simulink model "ThdRwLtStCshnFldTrgtPosSelc"  (R2018b)
settings: Solver=FixedStepDiscrete  StartTime=0.0  StopTime=10.0  RelTol=1e-3
undefined symbols (not defined in the file or in its folder): KeSMSw6sAcsEntryThdRwLtStCshnFldUpwdDnwdPos_Val, KeSMSw6sAcsEntryThdRwLtStCshnFldUpwdDnwdPosMax_Val, KeSMSw6sAcsEntryThdRwLtStCshnFldUpwdDnwdPosMin_Val, KeSMSw6sLugThdRwLtStCshnFldUpwdDnwdPos_Val, KeSMSw6sLugThdRwLtStCshnFldUpwdDnwdPosMax_Val, KeSMSw6sLugThdRwLtStCshnFldUpwdDnwdPosMin_Val, KeSMSwAcsEntryThdRwLtStCshnFldUpwdDnwdPos_Val, KeSMSwAcsEntryThdRwLtStCshnFldUpwdDnwdPosMax_Val, KeSMSwAcsEntryThdRwLtStCshnFldUpwdDnwdPosMin_Val, KeSMSwAcsMd32ThdRwLtFldUpwdDnwdPos_Val, KeSMSwAcsMd32ThdRwLtFldUpwdDnwdPosMax_Val, KeSMSwAcsMd32ThdRwLtFldUpwdDnwdPosMin_Val, KeSMSwLugThdRwLtStCshnFldUpwdDnwdPos_Val, KeSMSwLugThdRwLtStCshnFldUpwdDnwdPosMax_Val, KeSMSwLugThdRwLtStCshnFldUpwdDnwdPosMin_Val
libraries: TrgtPosSelcLib x4
settings Model: ModifiedHistory=2024.6.25 V2.1.0 557模式流程V1.6  Creator=sn2xws  LastModifiedBy=sn2xws
settings DataIOCC: SaveFormat=StructureWithTime
settings OptimizationCC: DefaultParameterBehavior=Inlined  EnhancedBackFolding=on  PassReuseOutputArgsAs=Individual arguments  ZeroExternalMemoryAtStartup=off  ZeroInternalMemoryAtStartup=off  OptimizeBlockOrder=speed  DifferentSizesBufferReuse=on  OptimizationCustomize=off
settings DebuggingCC: ParameterTunabilityLossMsg=error
settings SFSimCC: MATLABDynamicMemAlloc=off
settings RTWCC: SystemTargetFile=autosar.tlc  GenCodeOnly=on  TemplateMakefile=ert_default_tmf  Description=AUTOSAR  GenerateReport=on  IncludeHyperlinkInReport=on  LaunchReport=on  GenerateTraceInfo=on  GenerateTraceReport=on  GenerateTraceReportSl=on  GenerateTraceReportSf=on  GenerateTraceReportEml=on
settings CodeAppCC: ForceParamTrailComments=on  IgnoreCustomStorageClasses=off  OperatorAnnotations=on  SimulinkDataObjDesc=on  SFDataObjDesc=on  InsertBlockDesc=on
settings STFCustomTargetCC: TargetLangStandard=C99 (ISO)  MultiwordLength=256  ParMdlRefBuildCompliant=on  CompOptLevelCompliant=on  IncludeMdlTerminateFcn=off  CombineOutputUpdateFcns=on  SuppressErrorStatus=on  ERTCustomFileBanners=on  SupportNonFinite=off  SupportComplex=off  SupportContinuousTime=off  SupportNonInlinedSFcns=off  RemoveResetFunc=on  MATLABClassNameForMDSCustomization=Simulink.SoftwareTarget.ERTCustomization  AutosarCompliant=on  UseToolchainInfoCompliant=on  LookupTableObjectStructAxisOrder=2,1,3,4,...  LUTObjectStructOrderEvenSpacing=Size,Table,Breakpoints  SystemTargetFile=autosar.tlc
settings ERTTargetCC: TargetLangStandard=C99 (ISO)  ConcurrentExecutionCompliant=off  IncludeMdlTerminateFcn=off  SuppressErrorStatus=on  SupportNonFinite=off  SupportComplex=off  ModelStepFunctionPrototypeControlCompliant=off  CPPClassGenCompliant=off  AutosarCompliant=on  LookupTableObjectStructAxisOrder=2,1,3,4,...  LUTObjectStructOrderEvenSpacing=Size,Table,Breakpoints  InlinedParameterPlacement=NonHierarchical  ERTCustomFileTemplate=example_file_process.tlc  ERTFilePackagingFormat=Compact

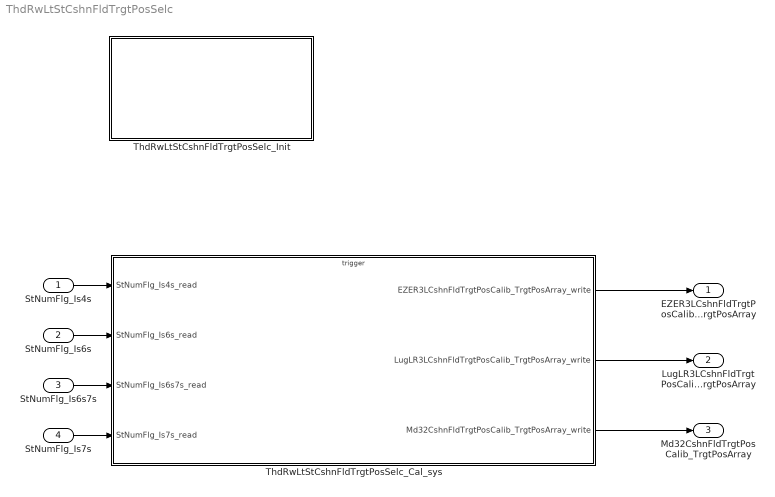
== system ThdRwLtStCshnFldTrgtPosSelc ==
  StNumFlg_Is4s : Inport  OutDataTypeStr=boolean  PortDimensions=1
  StNumFlg_Is6s : Inport  Port=2  OutDataTypeStr=boolean  PortDimensions=1
  StNumFlg_Is6s7s : Inport  Port=3  OutDataTypeStr=boolean  PortDimensions=1
  StNumFlg_Is7s : Inport  Port=4  OutDataTypeStr=boolean  PortDimensions=1
  ThdRwLtStCshnFldTrgtPosSelc_Cal_sys : Subsystem
  ThdRwLtStCshnFldTrgtPosSelc_Init : Subsystem
  EZER3LCshnFldTrgtPosCalib_TrgtPosArray : Outport  Description=|  OutDataTypeStr=uint16  PortDimensions=3
      | 0:Pos
      | 1:Max
      | 2:Min
  LugLR3LCshnFldTrgtPosCalib_TrgtPosArray : Outport  Description=|  Port=2  OutDataTypeStr=uint16  PortDimensions=3
      | 0:Pos
      | 1:Max
      | 2:Min
  Md32CshnFldTrgtPosCalib_TrgtPosArray : Outport  Description=|  Port=3  OutDataTypeStr=uint16  PortDimensions=3
      | 0:Pos
      | 1:Max
      | 2:Min
  wires:
  StNumFlg_Is4s/1 -> ThdRwLtStCshnFldTrgtPosSelc_Cal_sys/1(StNumFlg_Is4s_read)
  StNumFlg_Is6s/1 -> ThdRwLtStCshnFldTrgtPosSelc_Cal_sys/2(StNumFlg_Is6s_read)
  StNumFlg_Is6s7s/1 -> ThdRwLtStCshnFldTrgtPosSelc_Cal_sys/3(StNumFlg_Is6s7s_read)
  StNumFlg_Is7s/1 -> ThdRwLtStCshnFldTrgtPosSelc_Cal_sys/4(StNumFlg_Is7s_read)
  ThdRwLtStCshnFldTrgtPosSelc_Cal_sys/1(EZER3LCshnFldTrgtPosCalib_TrgtPosArray_write) -> EZER3LCshnFldTrgtPosCalib_TrgtPosArray/1
  ThdRwLtStCshnFldTrgtPosSelc_Cal_sys/2(LugLR3LCshnFldTrgtPosCalib_TrgtPosArray_write) -> LugLR3LCshnFldTrgtPosCalib_TrgtPosArray/1
  ThdRwLtStCshnFldTrgtPosSelc_Cal_sys/3(Md32CshnFldTrgtPosCalib_TrgtPosArray_write) -> Md32CshnFldTrgtPosCalib_TrgtPosArray/1

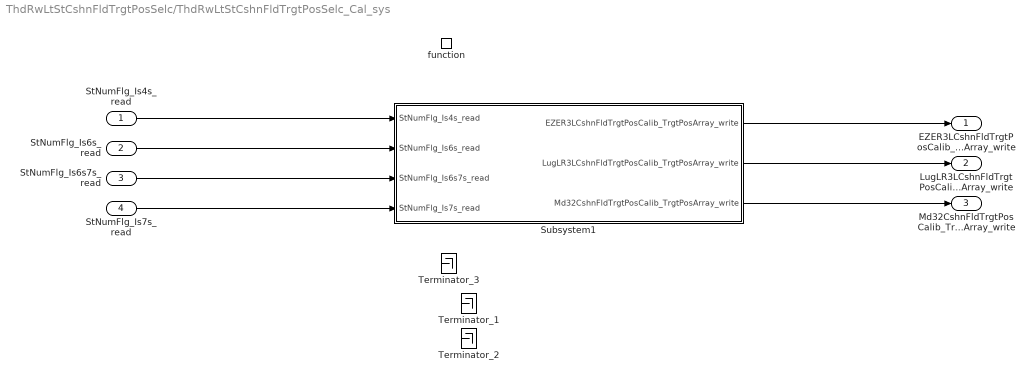
== system ThdRwLtStCshnFldTrgtPosSelc/ThdRwLtStCshnFldTrgtPosSelc_Cal_sys ==
  StNumFlg_Is4s_read : Inport
  StNumFlg_Is6s_read : Inport  Port=2
  StNumFlg_Is6s7s_read : Inport  Port=3
  StNumFlg_Is7s_read : Inport  Port=4
  function : TriggerPort  TriggerType=function-call  IsSimulinkFunction=on  FunctionName=ThdRwLtStCshnFldTrgtPosSelc_Cal  VariantControl=(inherit)
  Subsystem1 : Subsystem
  Terminator_1 : Terminator
  Terminator_2 : Terminator
  Terminator_3 : Terminator
  EZER3LCshnFldTrgtPosCalib_TrgtPosArray_write : Outport
      settings: EnsureOutportIsVirtual=on
  LugLR3LCshnFldTrgtPosCalib_TrgtPosArray_write : Outport  Port=2
      settings: EnsureOutportIsVirtual=on
  Md32CshnFldTrgtPosCalib_TrgtPosArray_write : Outport  Port=3
      settings: EnsureOutportIsVirtual=on
  wires:
  Subsystem1/1(EZER3LCshnFldTrgtPosCalib_TrgtPosArray_write) -> EZER3LCshnFldTrgtPosCalib_TrgtPosArray_write/1
  Subsystem1/2(LugLR3LCshnFldTrgtPosCalib_TrgtPosArray_write) -> LugLR3LCshnFldTrgtPosCalib_TrgtPosArray_write/1
  StNumFlg_Is4s_read/1 -> Subsystem1/1(StNumFlg_Is4s_read)
  StNumFlg_Is6s_read/1 -> Subsystem1/2(StNumFlg_Is6s_read)
  StNumFlg_Is6s7s_read/1 -> Subsystem1/3(StNumFlg_Is6s7s_read)
  StNumFlg_Is7s_read/1 -> Subsystem1/4(StNumFlg_Is7s_read)
  ? -> Terminator_1/1
  ? -> Terminator_2/1
  ? -> Terminator_3/1
  Subsystem1/3(Md32CshnFldTrgtPosCalib_TrgtPosArray_write) -> Md32CshnFldTrgtPosCalib_TrgtPosArray_write/1

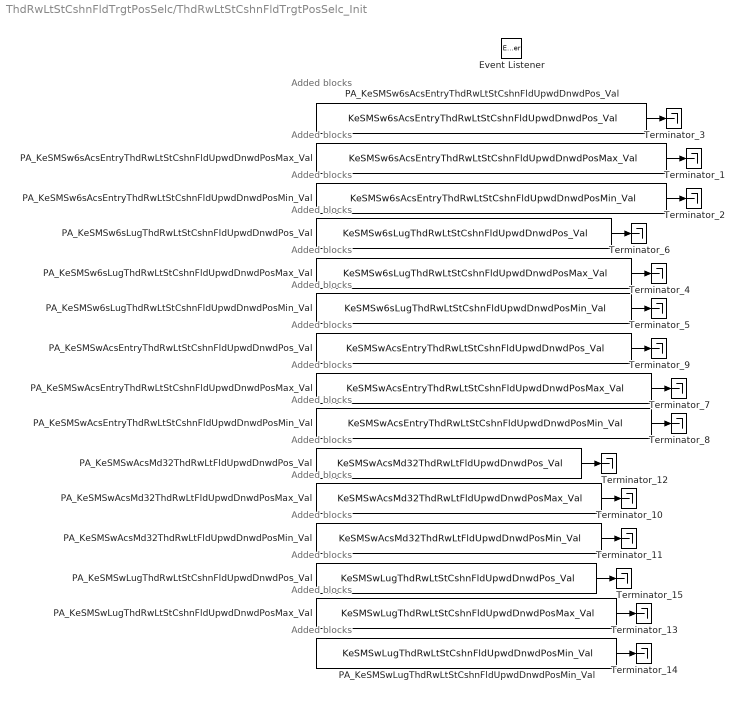
== system ThdRwLtStCshnFldTrgtPosSelc/ThdRwLtStCshnFldTrgtPosSelc_Init ==
  note: Added blocks
  note: Added blocks
  note: Added blocks
  note: Added blocks
  note: Added blocks
  note: Added blocks
  note: Added blocks
  note: Added blocks
  note: Added blocks
  note: Added blocks
  note: Added blocks
  note: Added blocks
  note: Added blocks
  note: Added blocks
  note: Added blocks
  Event Listener : EventListener  EventName=reset
  PA_KeSMSw6sAcsEntryThdRwLtStCshnFldUpwdDnwdPosMax_Val : Constant  Value=KeSMSw6sAcsEntryThdRwLtStCshnFldUpwdDnwdPosMax_Val
  PA_KeSMSw6sAcsEntryThdRwLtStCshnFldUpwdDnwdPosMin_Val : Constant  Value=KeSMSw6sAcsEntryThdRwLtStCshnFldUpwdDnwdPosMin_Val
  PA_KeSMSw6sAcsEntryThdRwLtStCshnFldUpwdDnwdPos_Val : Constant  Value=KeSMSw6sAcsEntryThdRwLtStCshnFldUpwdDnwdPos_Val
  PA_KeSMSw6sLugThdRwLtStCshnFldUpwdDnwdPosMax_Val : Constant  Value=KeSMSw6sLugThdRwLtStCshnFldUpwdDnwdPosMax_Val
  PA_KeSMSw6sLugThdRwLtStCshnFldUpwdDnwdPosMin_Val : Constant  Value=KeSMSw6sLugThdRwLtStCshnFldUpwdDnwdPosMin_Val
  PA_KeSMSw6sLugThdRwLtStCshnFldUpwdDnwdPos_Val : Constant  Value=KeSMSw6sLugThdRwLtStCshnFldUpwdDnwdPos_Val
  PA_KeSMSwAcsEntryThdRwLtStCshnFldUpwdDnwdPosMax_Val : Constant  Value=KeSMSwAcsEntryThdRwLtStCshnFldUpwdDnwdPosMax_Val
  PA_KeSMSwAcsEntryThdRwLtStCshnFldUpwdDnwdPosMin_Val : Constant  Value=KeSMSwAcsEntryThdRwLtStCshnFldUpwdDnwdPosMin_Val
  PA_KeSMSwAcsEntryThdRwLtStCshnFldUpwdDnwdPos_Val : Constant  Value=KeSMSwAcsEntryThdRwLtStCshnFldUpwdDnwdPos_Val
  PA_KeSMSwAcsMd32ThdRwLtFldUpwdDnwdPosMax_Val : Constant  Value=KeSMSwAcsMd32ThdRwLtFldUpwdDnwdPosMax_Val
  PA_KeSMSwAcsMd32ThdRwLtFldUpwdDnwdPosMin_Val : Constant  Value=KeSMSwAcsMd32ThdRwLtFldUpwdDnwdPosMin_Val
  PA_KeSMSwAcsMd32ThdRwLtFldUpwdDnwdPos_Val : Constant  Value=KeSMSwAcsMd32ThdRwLtFldUpwdDnwdPos_Val
  PA_KeSMSwLugThdRwLtStCshnFldUpwdDnwdPosMax_Val : Constant  Value=KeSMSwLugThdRwLtStCshnFldUpwdDnwdPosMax_Val
  PA_KeSMSwLugThdRwLtStCshnFldUpwdDnwdPosMin_Val : Constant  Value=KeSMSwLugThdRwLtStCshnFldUpwdDnwdPosMin_Val
  PA_KeSMSwLugThdRwLtStCshnFldUpwdDnwdPos_Val : Constant  Value=KeSMSwLugThdRwLtStCshnFldUpwdDnwdPos_Val
  Terminator_{1..15} (15 alike) : Terminator
  wires:
  PA_KeSMSw6sAcsEntryThdRwLtStCshnFldUpwdDnwdPosMax_Val/1 -> Terminator_1/1
  PA_KeSMSw6sAcsEntryThdRwLtStCshnFldUpwdDnwdPosMin_Val/1 -> Terminator_2/1
  PA_KeSMSw6sAcsEntryThdRwLtStCshnFldUpwdDnwdPos_Val/1 -> Terminator_3/1
  PA_KeSMSw6sLugThdRwLtStCshnFldUpwdDnwdPosMax_Val/1 -> Terminator_4/1
  PA_KeSMSw6sLugThdRwLtStCshnFldUpwdDnwdPosMin_Val/1 -> Terminator_5/1
  PA_KeSMSw6sLugThdRwLtStCshnFldUpwdDnwdPos_Val/1 -> Terminator_6/1
  PA_KeSMSwAcsEntryThdRwLtStCshnFldUpwdDnwdPosMax_Val/1 -> Terminator_7/1
  PA_KeSMSwAcsEntryThdRwLtStCshnFldUpwdDnwdPosMin_Val/1 -> Terminator_8/1
  PA_KeSMSwAcsEntryThdRwLtStCshnFldUpwdDnwdPos_Val/1 -> Terminator_9/1
  PA_KeSMSwAcsMd32ThdRwLtFldUpwdDnwdPosMax_Val/1 -> Terminator_10/1
  PA_KeSMSwAcsMd32ThdRwLtFldUpwdDnwdPosMin_Val/1 -> Terminator_11/1
  PA_KeSMSwAcsMd32ThdRwLtFldUpwdDnwdPos_Val/1 -> Terminator_12/1
  PA_KeSMSwLugThdRwLtStCshnFldUpwdDnwdPosMax_Val/1 -> Terminator_13/1
  PA_KeSMSwLugThdRwLtStCshnFldUpwdDnwdPosMin_Val/1 -> Terminator_14/1
  PA_KeSMSwLugThdRwLtStCshnFldUpwdDnwdPos_Val/1 -> Terminator_15/1

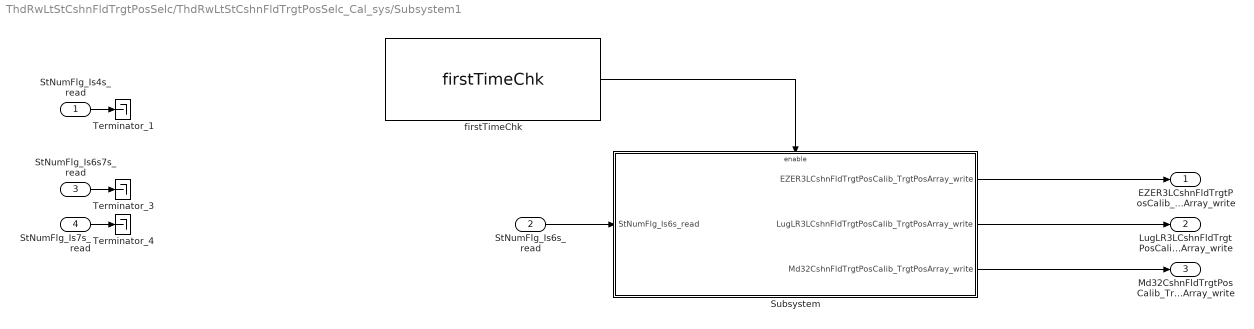
== system ThdRwLtStCshnFldTrgtPosSelc/ThdRwLtStCshnFldTrgtPosSelc_Cal_sys/Subsystem1 ==
  StNumFlg_Is4s_read : Inport
  StNumFlg_Is6s_read : Inport  Port=2
  StNumFlg_Is6s7s_read : Inport  Port=3
  StNumFlg_Is7s_read : Inport  Port=4
  Subsystem : Subsystem
  Terminator_1 : Terminator
  Terminator_3 : Terminator
  Terminator_4 : Terminator
  firstTimeChk : TrgtPosSelcLib/firstTimeChk  SystemSampleTime=-1
  EZER3LCshnFldTrgtPosCalib_TrgtPosArray_write : Outport
      settings: EnsureOutportIsVirtual=on
  LugLR3LCshnFldTrgtPosCalib_TrgtPosArray_write : Outport  Port=2
      settings: EnsureOutportIsVirtual=on
  Md32CshnFldTrgtPosCalib_TrgtPosArray_write : Outport  Port=3
      settings: EnsureOutportIsVirtual=on
  wires:
  StNumFlg_Is4s_read/1 -> Terminator_1/1
  StNumFlg_Is7s_read/1 -> Terminator_4/1
  StNumFlg_Is6s7s_read/1 -> Terminator_3/1
  StNumFlg_Is6s_read/1 -> Subsystem/1(StNumFlg_Is6s_read)
  firstTimeChk/1 -> Subsystem/Enable
  Subsystem/1(EZER3LCshnFldTrgtPosCalib_TrgtPosArray_write) -> EZER3LCshnFldTrgtPosCalib_TrgtPosArray_write/1
  Subsystem/2(LugLR3LCshnFldTrgtPosCalib_TrgtPosArray_write) -> LugLR3LCshnFldTrgtPosCalib_TrgtPosArray_write/1
  Subsystem/3(Md32CshnFldTrgtPosCalib_TrgtPosArray_write) -> Md32CshnFldTrgtPosCalib_TrgtPosArray_write/1

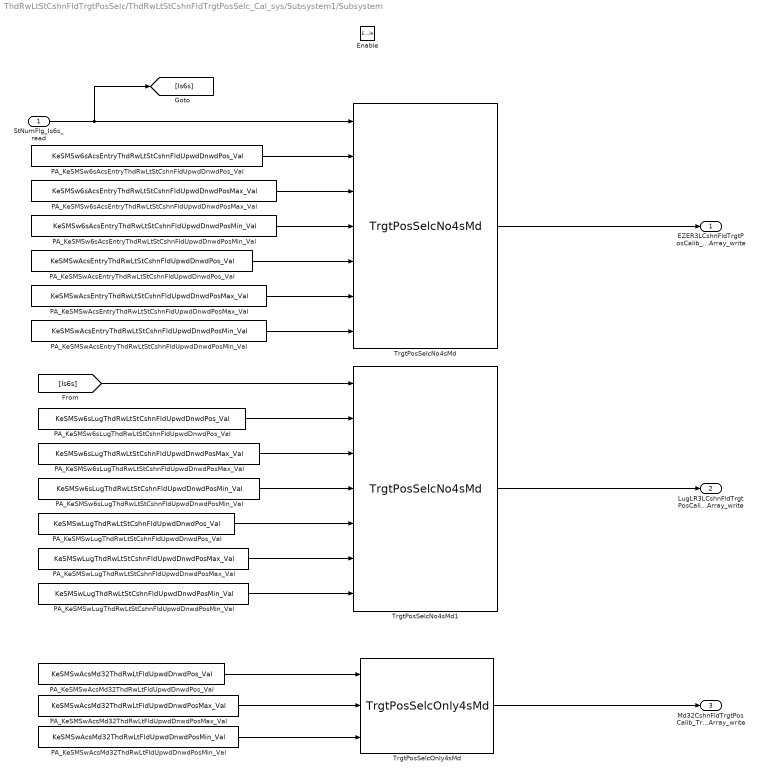
== system ThdRwLtStCshnFldTrgtPosSelc/ThdRwLtStCshnFldTrgtPosSelc_Cal_sys/Subsystem1/Subsystem ==
  StNumFlg_Is6s_read : Inport
  Enable : EnablePort
  PA_KeSMSw6sAcsEntryThdRwLtStCshnFldUpwdDnwdPosMax_Val : Constant  Value=KeSMSw6sAcsEntryThdRwLtStCshnFldUpwdDnwdPosMax_Val
  PA_KeSMSw6sAcsEntryThdRwLtStCshnFldUpwdDnwdPosMin_Val : Constant  Value=KeSMSw6sAcsEntryThdRwLtStCshnFldUpwdDnwdPosMin_Val
  PA_KeSMSw6sAcsEntryThdRwLtStCshnFldUpwdDnwdPos_Val : Constant  Value=KeSMSw6sAcsEntryThdRwLtStCshnFldUpwdDnwdPos_Val
  PA_KeSMSw6sLugThdRwLtStCshnFldUpwdDnwdPosMax_Val : Constant  Value=KeSMSw6sLugThdRwLtStCshnFldUpwdDnwdPosMax_Val
  PA_KeSMSw6sLugThdRwLtStCshnFldUpwdDnwdPosMin_Val : Constant  Value=KeSMSw6sLugThdRwLtStCshnFldUpwdDnwdPosMin_Val
  PA_KeSMSw6sLugThdRwLtStCshnFldUpwdDnwdPos_Val : Constant  Value=KeSMSw6sLugThdRwLtStCshnFldUpwdDnwdPos_Val
  PA_KeSMSwAcsEntryThdRwLtStCshnFldUpwdDnwdPosMax_Val : Constant  Value=KeSMSwAcsEntryThdRwLtStCshnFldUpwdDnwdPosMax_Val
  PA_KeSMSwAcsEntryThdRwLtStCshnFldUpwdDnwdPosMin_Val : Constant  Value=KeSMSwAcsEntryThdRwLtStCshnFldUpwdDnwdPosMin_Val
  PA_KeSMSwAcsEntryThdRwLtStCshnFldUpwdDnwdPos_Val : Constant  Value=KeSMSwAcsEntryThdRwLtStCshnFldUpwdDnwdPos_Val
  PA_KeSMSwAcsMd32ThdRwLtFldUpwdDnwdPosMax_Val : Constant  Value=KeSMSwAcsMd32ThdRwLtFldUpwdDnwdPosMax_Val
  PA_KeSMSwAcsMd32ThdRwLtFldUpwdDnwdPosMin_Val : Constant  Value=KeSMSwAcsMd32ThdRwLtFldUpwdDnwdPosMin_Val
  PA_KeSMSwAcsMd32ThdRwLtFldUpwdDnwdPos_Val : Constant  Value=KeSMSwAcsMd32ThdRwLtFldUpwdDnwdPos_Val
  PA_KeSMSwLugThdRwLtStCshnFldUpwdDnwdPosMax_Val : Constant  Value=KeSMSwLugThdRwLtStCshnFldUpwdDnwdPosMax_Val
  PA_KeSMSwLugThdRwLtStCshnFldUpwdDnwdPosMin_Val : Constant  Value=KeSMSwLugThdRwLtStCshnFldUpwdDnwdPosMin_Val
  PA_KeSMSwLugThdRwLtStCshnFldUpwdDnwdPos_Val : Constant  Value=KeSMSwLugThdRwLtStCshnFldUpwdDnwdPos_Val
  TrgtPosSelcNo4sMd : TrgtPosSelcLib/TrgtPosSelcNo4sMd  SystemSampleTime=-1
  TrgtPosSelcNo4sMd1 : TrgtPosSelcLib/TrgtPosSelcNo4sMd  SystemSampleTime=-1
  TrgtPosSelcOnly4sMd : TrgtPosSelcLib/TrgtPosSelcOnly4sMd  SystemSampleTime=-1
  EZER3LCshnFldTrgtPosCalib_TrgtPosArray_write : Outport
      settings: EnsureOutportIsVirtual=on
  LugLR3LCshnFldTrgtPosCalib_TrgtPosArray_write : Outport  Port=2
      settings: EnsureOutportIsVirtual=on
  Md32CshnFldTrgtPosCalib_TrgtPosArray_write : Outport  Port=3
      settings: EnsureOutportIsVirtual=on
  wires:
  StNumFlg_Is6s_read/1 -> [Is6s], TrgtPosSelcNo4sMd/1
  TrgtPosSelcNo4sMd1/1 -> LugLR3LCshnFldTrgtPosCalib_TrgtPosArray_write/1
  TrgtPosSelcNo4sMd/1 -> EZER3LCshnFldTrgtPosCalib_TrgtPosArray_write/1
  PA_KeSMSw6sAcsEntryThdRwLtStCshnFldUpwdDnwdPosMax_Val/1 -> TrgtPosSelcNo4sMd/3
  PA_KeSMSw6sAcsEntryThdRwLtStCshnFldUpwdDnwdPosMin_Val/1 -> TrgtPosSelcNo4sMd/4
  PA_KeSMSw6sAcsEntryThdRwLtStCshnFldUpwdDnwdPos_Val/1 -> TrgtPosSelcNo4sMd/2
  [Is6s] -> TrgtPosSelcNo4sMd1/1
  PA_KeSMSw6sLugThdRwLtStCshnFldUpwdDnwdPosMin_Val/1 -> TrgtPosSelcNo4sMd1/4
  PA_KeSMSw6sLugThdRwLtStCshnFldUpwdDnwdPosMax_Val/1 -> TrgtPosSelcNo4sMd1/3
  PA_KeSMSw6sLugThdRwLtStCshnFldUpwdDnwdPos_Val/1 -> TrgtPosSelcNo4sMd1/2
  PA_KeSMSwAcsEntryThdRwLtStCshnFldUpwdDnwdPosMax_Val/1 -> TrgtPosSelcNo4sMd/6
  PA_KeSMSwAcsEntryThdRwLtStCshnFldUpwdDnwdPosMin_Val/1 -> TrgtPosSelcNo4sMd/7
  PA_KeSMSwAcsEntryThdRwLtStCshnFldUpwdDnwdPos_Val/1 -> TrgtPosSelcNo4sMd/5
  PA_KeSMSwLugThdRwLtStCshnFldUpwdDnwdPosMax_Val/1 -> TrgtPosSelcNo4sMd1/6
  PA_KeSMSwLugThdRwLtStCshnFldUpwdDnwdPosMin_Val/1 -> TrgtPosSelcNo4sMd1/7
  PA_KeSMSwLugThdRwLtStCshnFldUpwdDnwdPos_Val/1 -> TrgtPosSelcNo4sMd1/5
  PA_KeSMSwAcsMd32ThdRwLtFldUpwdDnwdPos_Val/1 -> TrgtPosSelcOnly4sMd/1
  PA_KeSMSwAcsMd32ThdRwLtFldUpwdDnwdPosMax_Val/1 -> TrgtPosSelcOnly4sMd/2
  PA_KeSMSwAcsMd32ThdRwLtFldUpwdDnwdPosMin_Val/1 -> TrgtPosSelcOnly4sMd/3
  TrgtPosSelcOnly4sMd/1 -> Md32CshnFldTrgtPosCalib_TrgtPosArray_write/1
